simulink model "DynamiqueElectroaimants"  (R2018b)
settings: Solver=VariableStepAuto  StartTime=0.0  StopTime=10.0  RelTol=1e-3
values from neighbouring files (symbols this model uses):
  ae0 = 1    [Modele.m]
  ae1 = 1    [Modele.m]
  ae2 = 1    [Modele.m]
  ae3 = 1    [Modele.m]
  as0 = 1    [Modele.m]
  as1 = 1    [Modele.m]
  as2 = 1    [Modele.m]
  as3 = 1    [Modele.m]
  be1 = 1    [Modele.m]
  XA = r_abc    (= 0.0952)    [Modele.m]
  XB = -r_abc*sind(30)    [Modele.m]
  XC = -r_abc*sind(30)    [Modele.m]
  YA = 0    [Modele.m]
  YB = r_abc*cosd(30)    [Modele.m]
  YC = -r_abc*cosd(30)    [Modele.m]
settings Model: Creator=Vincent  LastModifiedBy=Vincent

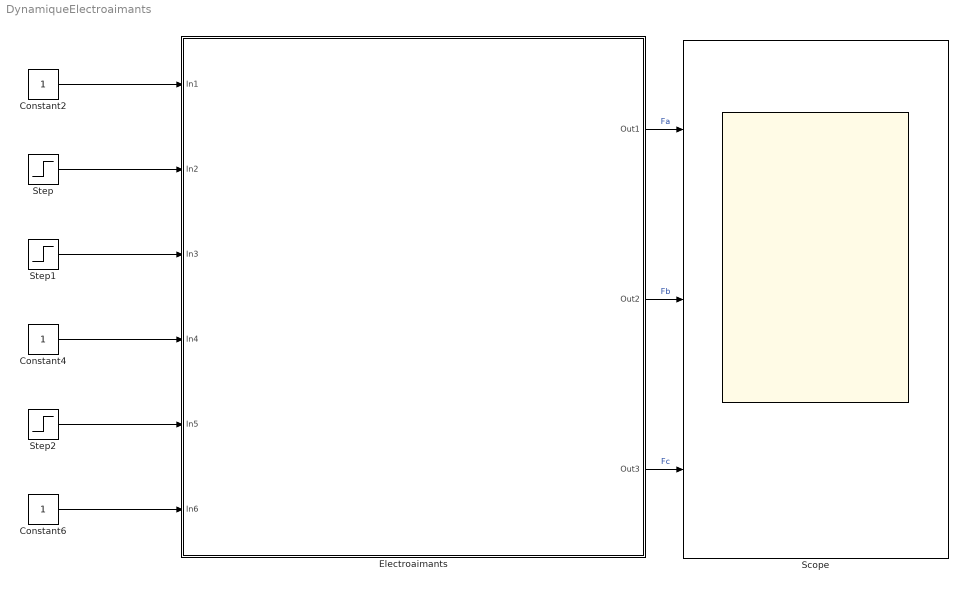
== system DynamiqueElectroaimants ==
  Constant2 : Constant
  Constant4 : Constant
  Constant6 : Constant
  Electroaimants : Subsystem
  Scope : Scope  NumInputPorts=3
  Step : Step  SampleTime=0
  Step1 : Step  SampleTime=0
  Step2 : Step  SampleTime=0
  wires:
  Constant2/1 -> Electroaimants/1(In1)
  Step/1 -> Electroaimants/2(In2)
  Step1/1 -> Electroaimants/3(In3)
  Constant4/1 -> Electroaimants/4(In4)
  Step2/1 -> Electroaimants/5(In5)
  Constant6/1 -> Electroaimants/6(In6)
  Electroaimants/1(Out1) -> Scope/1  "Fa"
  Electroaimants/2(Out2) -> Scope/2  "Fb"
  Electroaimants/3(Out3) -> Scope/3  "Fc"

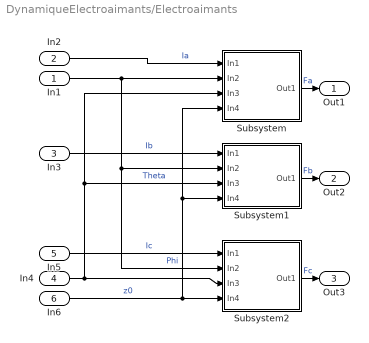
== system DynamiqueElectroaimants/Electroaimants ==
  In1 : Inport
  In2 : Inport  Port=2
  In3 : Inport  Port=3
  In4 : Inport  Port=4
  In5 : Inport  Port=5
  In6 : Inport  Port=6
  Subsystem : Subsystem
  Subsystem1 : Subsystem
  Subsystem2 : Subsystem
  Out1 : Outport
  Out2 : Outport  Port=2
  Out3 : Outport  Port=3
  wires:
  In6/1 -> Subsystem2/4(In4), Subsystem1/4(In4), Subsystem/4(In4)  "z0"
  In4/1 -> Subsystem2/3(In3), Subsystem/3(In3), Subsystem1/3(In3)  "Theta"
  In5/1 -> Subsystem2/1(In1)  "Ic"
  In1/1 -> Subsystem/2(In2), Subsystem2/2(In2), Subsystem1/2(In2)  "Phi"
  Subsystem2/1(Out1) -> Out3/1  "Fc"
  In2/1 -> Subsystem/1(In1)  "Ia"
  In3/1 -> Subsystem1/1(In1)  "Ib"
  Subsystem1/1(Out1) -> Out2/1  "Fb"
  Subsystem/1(Out1) -> Out1/1  "Fa"

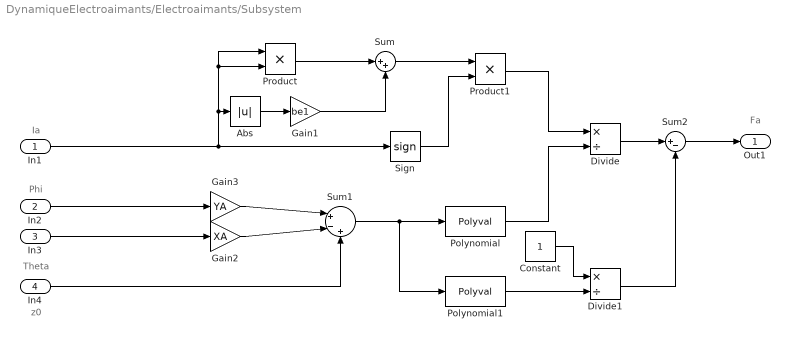
== system DynamiqueElectroaimants/Electroaimants/Subsystem ==
  note: Fa
  note: z0
  note: Theta
  note: Phi
  note: Ia
  In1 : Inport
  In2 : Inport  Port=2
  In3 : Inport  Port=3
  In4 : Inport  Port=4
  Abs : Abs
  Constant : Constant
  Divide : Product  Inputs=*/
  Divide1 : Product  Inputs=*/
  Gain1 : Gain  Gain=be1
  Gain2 : Gain  Gain=XA
  Gain3 : Gain  Gain=YA
  Polynomial : Polyval  Coefs=[ae3 ae2 ae1 ae0]
  Polynomial1 : Polyval  Coefs=[as3 as2 as1 as0]
  Product : Product
  Product1 : Product
  Sign : Signum
  Sum : Sum  Inputs=|++
  Sum1 : Sum  Inputs=|+-+
  Sum2 : Sum  Inputs=|+-
  Out1 : Outport
  wires:
  Sum/1 -> Product1/1
  Product1/1 -> Divide/1
  Gain2/1 -> Sum1/2
  Sum2/1 -> Out1/1
  Constant/1 -> Divide1/1
  Product/1 -> Sum/1
  Polynomial/1 -> Divide/2
  In1/1 -> Product/1, Product/2, Abs/1, Sign/1
  Abs/1 -> Gain1/1
  Gain1/1 -> Sum/2
  Polynomial1/1 -> Divide1/2
  Sum1/1 -> Polynomial1/1, Polynomial/1
  Sign/1 -> Product1/2
  In4/1 -> Sum1/3
  Divide/1 -> Sum2/1
  Gain3/1 -> Sum1/1
  Divide1/1 -> Sum2/2
  In2/1 -> Gain3/1
  In3/1 -> Gain2/1

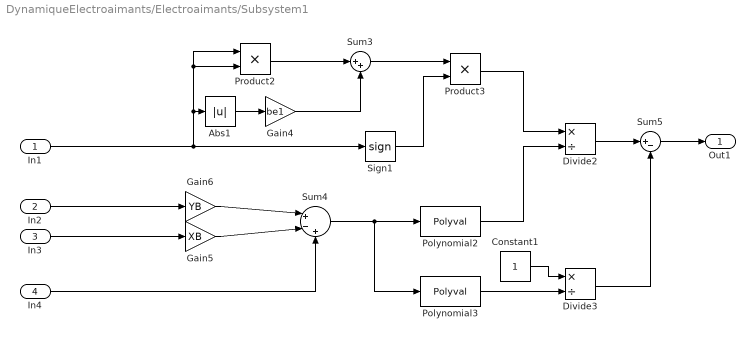
== system DynamiqueElectroaimants/Electroaimants/Subsystem1 ==
  In1 : Inport
  In2 : Inport  Port=2
  In3 : Inport  Port=3
  In4 : Inport  Port=4
  Abs1 : Abs
  Constant1 : Constant
  Divide2 : Product  Inputs=*/
  Divide3 : Product  Inputs=*/
  Gain4 : Gain  Gain=be1
  Gain5 : Gain  Gain=XB
  Gain6 : Gain  Gain=YB
  Polynomial2 : Polyval  Coefs=[ae3 ae2 ae1 ae0]
  Polynomial3 : Polyval  Coefs=[as3 as2 as1 as0]
  Product2 : Product
  Product3 : Product
  Sign1 : Signum
  Sum3 : Sum  Inputs=|++
  Sum4 : Sum  Inputs=|+-+
  Sum5 : Sum  Inputs=|+-
  Out1 : Outport
  wires:
  In2/1 -> Gain6/1
  Gain6/1 -> Sum4/1
  In4/1 -> Sum4/3
  Gain5/1 -> Sum4/2
  Sum4/1 -> Polynomial3/1, Polynomial2/1
  In1/1 -> Product2/1, Product2/2, Abs1/1, Sign1/1
  Constant1/1 -> Divide3/1
  Sign1/1 -> Product3/2
  Divide2/1 -> Sum5/1
  In3/1 -> Gain5/1
  Divide3/1 -> Sum5/2
  Polynomial3/1 -> Divide3/2
  Product3/1 -> Divide2/1
  Gain4/1 -> Sum3/2
  Abs1/1 -> Gain4/1
  Product2/1 -> Sum3/1
  Sum3/1 -> Product3/1
  Polynomial2/1 -> Divide2/2
  Sum5/1 -> Out1/1

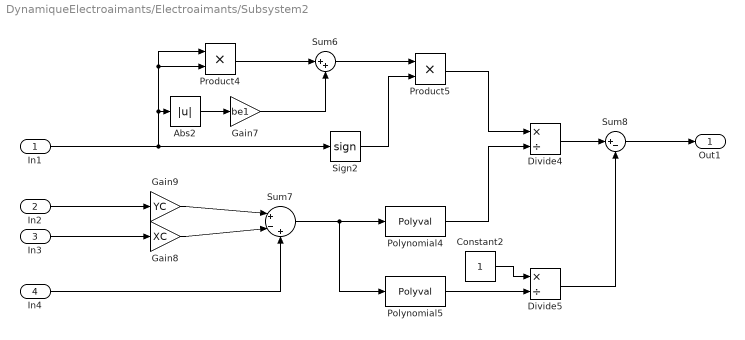
== system DynamiqueElectroaimants/Electroaimants/Subsystem2 ==
  In1 : Inport
  In2 : Inport  Port=2
  In3 : Inport  Port=3
  In4 : Inport  Port=4
  Abs2 : Abs
  Constant2 : Constant
  Divide4 : Product  Inputs=*/
  Divide5 : Product  Inputs=*/
  Gain7 : Gain  Gain=be1
  Gain8 : Gain  Gain=XC
  Gain9 : Gain  Gain=YC
  Polynomial4 : Polyval  Coefs=[ae3 ae2 ae1 ae0]
  Polynomial5 : Polyval  Coefs=[as3 as2 as1 as0]
  Product4 : Product
  Product5 : Product
  Sign2 : Signum
  Sum6 : Sum  Inputs=|++
  Sum7 : Sum  Inputs=|+-+
  Sum8 : Sum  Inputs=|+-
  Out1 : Outport
  wires:
  Gain9/1 -> Sum7/1
  Gain8/1 -> Sum7/2
  Divide5/1 -> Sum8/2
  Divide4/1 -> Sum8/1
  Constant2/1 -> Divide5/1
  In1/1 -> Product4/1, Product4/2, Abs2/1, Sign2/1
  Sum7/1 -> Polynomial5/1, Polynomial4/1
  Sign2/1 -> Product5/2
  In2/1 -> Gain9/1
  Product4/1 -> Sum6/1
  Product5/1 -> Divide4/1
  In4/1 -> Sum7/3
  Polynomial5/1 -> Divide5/2
  Gain7/1 -> Sum6/2
  Polynomial4/1 -> Divide4/2
  Sum6/1 -> Product5/1
  Abs2/1 -> Gain7/1
  Sum8/1 -> Out1/1
  In3/1 -> Gain8/1
